simulink model "Quadcopter_Hinfinity_Discrete"  (R2016b)
settings: Solver=ode45  StartTime=0.0  StopTime=33  RelTol=1e-3  EnableMultiTasking=on
undefined symbols (not defined in the file): A, B, C, D, K1d, sigbuilder_block, Ts, X0
libraries: simulink x1
settings Model: Creator=Toshiba  LastModifiedBy=AAstudillo
settings DataIOCC: LimitDataPoints=on  SaveFormat=Array  SignalLoggingSaveFormat=ModelDataLogs
settings OptimizationCC: LifeSpan=inf
settings DebuggingCC: SolverPrmCheckMsg=warning  MultiTaskDSMMsg=warning  MultiTaskCondExecSysMsg=none  SFUnexpectedBacktrackingDiag=warning  SFNoUnconditionalDefaultTransitionDiag=warning  SFExecutionAtInitializationDiag=none
settings HardwareCC: ProdBitPerPointer=32  ProdBitPerSizeT=32  ProdBitPerPtrDiffT=32  ProdLargestAtomicFloat=None  ProdIntDivRoundTo=Undefined  ProdEndianess=Unspecified  ProdWordSize=32  ProdHWDeviceType=32-bit Generic
settings ModelReferenceCC: PropagateSignalLabelsOutOfModel=off
settings GRTTargetCC: TargetLangStandard=C89/C90 (ANSI)  GeneratePreprocessorConditionals=Disable all
settings ConfigComp: CovMetricSettings=dw  CovHtmlReporting=on  CovSaveCumulativeToWorkspaceVar=on  CovSaveSingleToWorkspaceVar=on  CovExternalEMLEnable=off

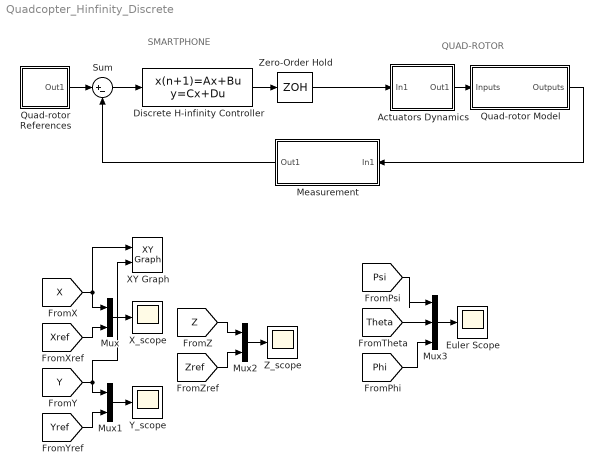
== system Quadcopter_Hinfinity_Discrete ==
  note: QUAD-ROTOR
  note: SMARTPHONE
  Actuators Dynamics : Subsystem
  Discrete H-infinity Controller : DiscreteStateSpace  A=K1d.A  B=K1d.B  C=K1d.C  D=K1d.D  X0=zeros(size(K1d.A,1),1)  SampleTime=Ts
  Euler Scope : Scope
  Measurement : Subsystem
  Mux : Mux  Inputs=2
  Mux1 : Mux  Inputs=2
  Mux2 : Mux  Inputs=2
  Mux3 : Mux  Inputs=3
  Quad-rotor Model : Subsystem
  Quad-rotor References : Subsystem
  Sum : Sum  Inputs=|+-
  XY Graph : simulink/Sinks/XY Graph  xmin=-1  xmax=1  ymin=-1  ymax=1  st=-1
  X_scope : Scope
  Y_scope : Scope
  Z_scope : Scope
  Zero-Order Hold : ZeroOrderHold  SampleTime=Ts
  wires:
  Quad-rotor References/1(Out1) -> Sum/1
  Mux/1 -> X_scope/1
  Mux1/1 -> Y_scope/1
  Mux2/1 -> Z_scope/1
  [X] -> Mux/1, XY Graph/1
  [Xref] -> Mux/2
  [Y] -> Mux1/1, XY Graph/2
  [Yref] -> Mux1/2
  [Z] -> Mux2/1
  [Zref] -> Mux2/2
  Actuators Dynamics/1(Out1) -> Quad-rotor Model/1(Inputs)
  Sum/1 -> Discrete H-infinity Controller/1
  Discrete H-infinity Controller/1 -> Zero-Order Hold/1
  Zero-Order Hold/1 -> Actuators Dynamics/1(In1)
  Measurement/1(Out1) -> Sum/2
  Quad-rotor Model/1(Outputs) -> Measurement/1(In1)
  [Psi] -> Mux3/1
  Mux3/1 -> Euler Scope/1
  [Theta] -> Mux3/2
  [Phi] -> Mux3/3

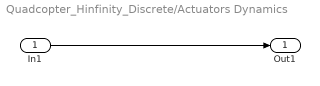
== system Quadcopter_Hinfinity_Discrete/Actuators Dynamics ==
  In1 : Inport
  Out1 : Outport
  wires:
  In1/1 -> Out1/1

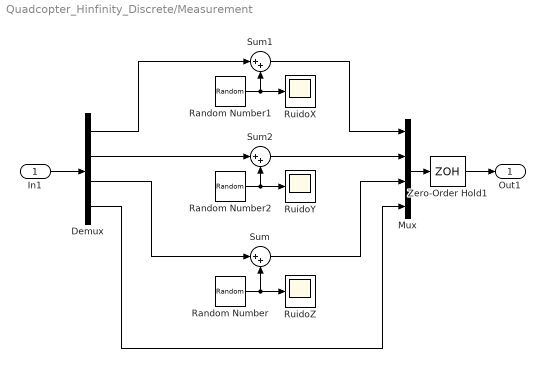
== system Quadcopter_Hinfinity_Discrete/Measurement ==
  In1 : Inport
  Demux : Demux
  Mux : Mux
  Random Number : RandomNumber  Variance=0.04  SampleTime=Ts
  Random Number1 : RandomNumber  Variance=0.001  SampleTime=Ts
  Random Number2 : RandomNumber  Variance=0.001  SampleTime=Ts
  RuidoX : Scope
  RuidoY : Scope
  RuidoZ : Scope
  Sum : Sum  Inputs=|++
  Sum1 : Sum  Inputs=|++
  Sum2 : Sum  Inputs=|++
  Zero-Order Hold1 : ZeroOrderHold  SampleTime=Ts
  Out1 : Outport
  wires:
  Zero-Order Hold1/1 -> Out1/1
  Mux/1 -> Zero-Order Hold1/1
  Random Number/1 -> Sum/2, RuidoZ/1
  Demux/4 -> Mux/4
  Demux/3 -> Sum/1
  Sum/1 -> Mux/3
  Demux/1 -> Sum1/1
  Sum1/1 -> Mux/1
  Random Number2/1 -> RuidoY/1, Sum2/2
  Demux/2 -> Sum2/1
  Sum2/1 -> Mux/2
  Random Number1/1 -> RuidoX/1, Sum1/2
  In1/1 -> Demux/1

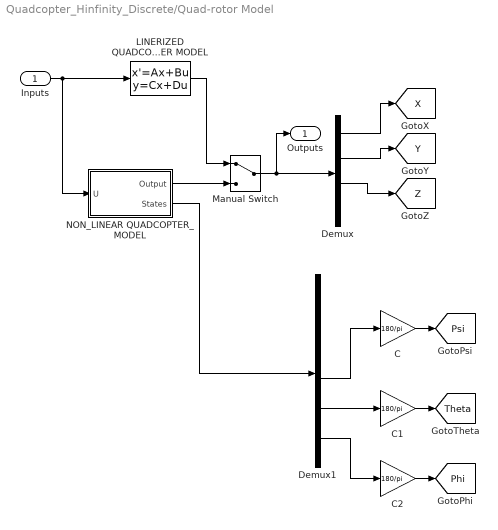
== system Quadcopter_Hinfinity_Discrete/Quad-rotor Model ==
  Inputs : Inport
  C : Gain  Gain=180/pi
  C1 : Gain  Gain=180/pi
  C2 : Gain  Gain=180/pi
  Demux : Demux
  Demux1 : Demux  Outputs=12
  LINERIZED QUADCOPTER MODEL : StateSpace  A=A  B=B  C=C  D=D  X0=X0
  Manual Switch : ManualSwitch
  NON_LINEAR QUADCOPTER_MODEL : Subsystem
  Outputs : Outport
  tag scope: Phi=global, Psi=global, Theta=global, X=global, Y=global, Z=global
  wires:
  Inputs/1 -> LINERIZED QUADCOPTER MODEL/1, NON_LINEAR QUADCOPTER_MODEL/1(U)
  LINERIZED QUADCOPTER MODEL/1 -> Manual Switch/1
  Manual Switch/1 -> Outputs/1, Demux/1
  NON_LINEAR QUADCOPTER_MODEL/1("Output ") -> Manual Switch/2
  Demux/3 -> [Z]
  Demux/2 -> [Y]
  Demux/1 -> [X]
  NON_LINEAR QUADCOPTER_MODEL/2(States) -> Demux1/1
  C/1 -> [Psi]
  Demux1/7 -> C/1
  C1/1 -> [Theta]
  C2/1 -> [Phi]
  Demux1/9 -> C1/1
  Demux1/11 -> C2/1

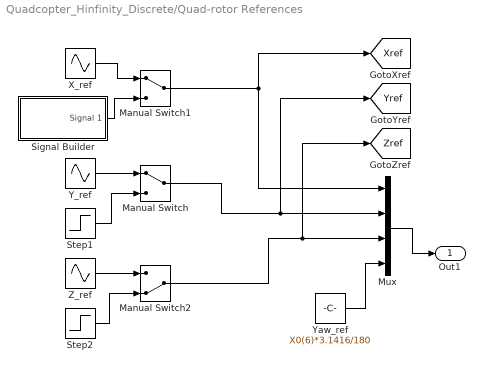
== system Quadcopter_Hinfinity_Discrete/Quad-rotor References ==
  Manual Switch : ManualSwitch
  Manual Switch1 : ManualSwitch
  Manual Switch2 : ManualSwitch  CurrentSetting=0
  Mux : Mux
  Signal Builder : Subsystem  Tag=STV Subsys  LoadFcn=sigbuilder_block('load');  StartFcn=sigbuilder_block('start');  StopFcn=sigbuilder_block('stop');  ClipboardFcn=sigbuilder_block('clipboard');  mask(Sigbuilder block){tuvar=[0:10]}
      mask help: Simulink:masks:SigbuilderBlock_MD
      mask init:
      | if ~strcmp(get_param(bdroot(gcbh),'SimulationStatus'),'stopped') tuvar = sigbuilder_block('maskInit'); end
      settings: CopyFcn=sigbuilder_block('copy');  DeleteFcn=sigbuilder_block('delete');  ModelCloseFcn=sigbuilder_block('modelClose');  PreSaveFcn=sigbuilder_block('preSave');  PauseFcn=sigbuilder_block('pause');  ContinueFcn=sigbuilder_block('continue');  NameChangeFcn=sigbuilder_block('namechange');  OpenFcn=sigbuilder_block('open',[6 30 1012.5 447.75 ]);  CloseFcn=sigbuilder_block('close');
      mask Display: plot(0, 0, 100, 100,[2, 2, 32, 32, 2], [68, 8, 8, 68, 68],[32, 2], [38, 38], [32, 19, 2],[53, 60, 44], [32, 17, 17, 2],[16, 16, 31, 31]);txt = getActiveGroup(gcbh);text(2, 100, txt,'verticalAlignment', 'top');
  Step1 : Step  Time=20  Before=1  After=0  SampleTime=0
  Step2 : Step  Time=20  Before=1  After=2  SampleTime=0
  X_ref : Sin  Frequency=3.141592654*0.1  SampleTime=0
  Y_ref : Sin  Frequency=3.141592654*0.1  Phase=3.141592654/2  SampleTime=0
  Yaw_ref : Constant  Value=X0(6)*3.1416/180
  Z_ref : Sin  Bias=1  Frequency=3.141592654*0.05  Phase=3.141592654  SampleTime=0
  Out1 : Outport
  tag scope: Xref=global, Yref=global, Zref=global
  wires:
  Mux/1 -> Out1/1
  Yaw_ref/1 -> Mux/4
  X_ref/1 -> Manual Switch1/1
  Manual Switch1/1 -> [Xref], Mux/1
  Signal Builder/1(Signal 1) -> Manual Switch1/2
  Y_ref/1 -> Manual Switch/1
  Step1/1 -> Manual Switch/2
  Manual Switch/1 -> [Yref], Mux/2
  Step2/1 -> Manual Switch2/2
  Z_ref/1 -> Manual Switch2/1
  Manual Switch2/1 -> [Zref], Mux/3

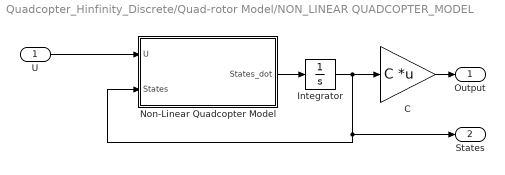
== system Quadcopter_Hinfinity_Discrete/Quad-rotor Model/NON_LINEAR QUADCOPTER_MODEL ==
  U : Inport
  C : Gain  Gain=C  Multiplication=Matrix(K*u)
  Integrator : Integrator  InitialCondition=X0
  Non-Linear Quadcopter Model : MATLAB Function  TreatAsAtomicUnit=on
  "Output " : Outport
  States : Outport  Port=2
  wires:
  Non-Linear Quadcopter Model/1(States_dot) -> Integrator/1
  Integrator/1 -> Non-Linear Quadcopter Model/2(States), States/1, C/1
  U/1 -> Non-Linear Quadcopter Model/1(U)
  C/1 -> "Output "/1

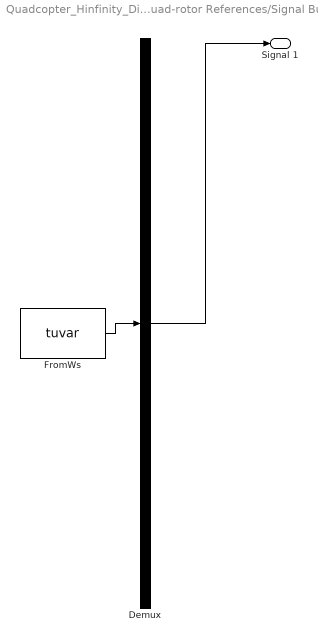
== system Quadcopter_Hinfinity_Discrete/Quad-rotor References/Signal Builder ==
  Demux : Demux  Tag=STV Demux  Outputs=1
  FromWs : FromWorkspace  Tag=STV FromWs  VariableName=tuvar  SampleTime=0
      SigBuilderData=|
      | common.afterFinalStr = 'Extrapolate'
      | common.sampleTime = 0
      | dataSet.timeRange = [0 30]
      | dataSet.name = 'Group 1'
      | sbobj.Groups.Name = 'Group 1'
      | sbobj.Groups.Signals.Name = 'Signal 1'
      | sbobj.Groups.Signals.XData = [0 4 5 6 10 10 30]
      | sbobj.Groups.Signals.YData = [0 0 0.14 0.48 0.925 0.99 0.99]
      | sbobj.Groups.TimeRange = [0 30]
  Signal 1 : Outport  Tag=STV Outport
  wires:
  Demux/1 -> Signal 1/1
  FromWs/1 -> Demux/1

== matlab function Quadcopter_Hinfinity_Discrete/Quad-rotor Model/NON_LINEAR QUADCOPTER_MODEL/Non-Linear Quadcopter Model ==
  data: U input; States input; States_dot output
function States_dot  = fcn(U, States)

% Gravity constant
              g = 9.807;

              m = 1.568;
              Ixx = 0.0135;
              Iyy = 0.0124;
              Izz = 0.0336;

    %Inputs = U, States
    %Outputs = States_dot  
    %States: X dX Y dY Z dZ Psi dPsi Theta dTheta Phi dPhi
    %        1  2 3  4 5  6  7   8     9      10   11  12
    
    U1 = U(1);
    U2 = U(2);
    U3 = U(3);
    U4 = U(4);

    dX = States(2);
    %ddX = ((U1/m)*sin(States(9))) + g*sin(States(9));
    %ddX = (U1/m)*(cos(States(7))*sin(States(9))*cos(States(11)) + sin(States(7))*sin(States(11)));
    ddX = -States(10)*States(6) + States(8)*States(4) + g*sin(States(9));
    dY = States(4);
    %ddY = ((U1/m)*cos(States(9))*sin(States(11))) + g*cos(States(9))*sin(States(11));
    %ddY = (U1/m)*(sin(States(7))*sin(States(9))*cos(States(11)) - cos(States(7))*sin(States(11)));
    ddY = States(8)*States(2) - States(12)*States(6) + g*cos(States(9))*sin(States(11));
    dZ = States(6);
    %ddZ = ((U1/m)*cos(States(9))*cos(States(11))) + (g*cos(States(9))*cos(States(11))) - g;
    %ddZ = (((U1+m*g)/m)*cos(States(9))*cos(States(11))) - g;
    ddZ = States(10)*States(2) - States(12)*States(4) - g*cos(States(9))*cos(States(11)) + (U1+m*g)/m;
    
    dPsi = States(8);
    ddPsi = (((Ixx-Iyy)/Izz)*States(12)*States(10)) + (U2/Izz);
    dTheta = States(10);
    ddTheta = (((Izz-Ixx)/Iyy)*States(12)*States(8)) + (U3/Iyy);
    dPhi = States(12);
    ddPhi = (((Iyy-Izz)/Ixx)*States(10)*States(8)) + (U4/Ixx);


States_dot = [dX, ddX, dY, ddY, dZ, ddZ, dPsi, ddPsi, dTheta, ddTheta, dPhi, ddPhi]';
